simulink model "simpleDemo"  (R2024a)
settings: Solver=VariableStepAuto  StartTime=0.0  StopTime=10.0  RelTol=1e-3
values from neighbouring files (symbols this model uses):
  pathC = 1    [sampleDD.sldd]
settings Model: DataDictionary=sampleDD.sldd  Creator=ntyler  LastModifiedBy=ntyler

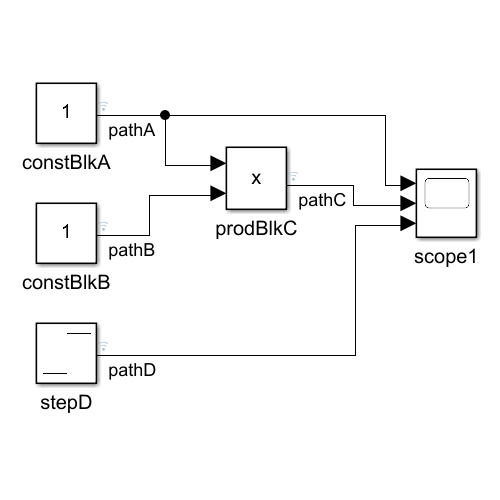
[thumbnail: Simulink's stored preview of the top-level diagram]
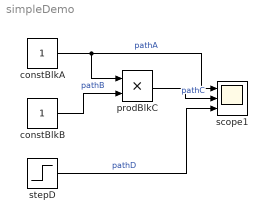
== system simpleDemo ==
  constBlkA : Constant  OutMin=0  OutMax=100  OutDataTypeStr=single  SampleTime=-1
  constBlkB : Constant  OutMin=0  OutMax=100  OutDataTypeStr=single  SampleTime=-1
  prodBlkC : Product  OutMin=pathC.Min  OutMax=pathC.Max  OutDataTypeStr=pathC.DataType
  scope1 : Scope  NumInputPorts=3
  stepD : Step  SampleTime=0
  wires:
  constBlkA/1 -> prodBlkC/1, scope1/1  "pathA"
  constBlkB/1 -> prodBlkC/2  "pathB"
  prodBlkC/1 -> scope1/2  "pathC"
  stepD/1 -> scope1/3  "pathD"
